simulink model "GlowPlug_harness"  (Simulink 7.7)
settings: Solver=FixedStepDiscrete  SolverMode=SingleTasking  StartTime=0.0  StopTime=100  FixedStep=0.1  RelTol=1e-3
InitFcn:
  | if signalbuilder('GlowPlug_harness/Signal_Builder','activegroup') == 1
  |   CD_GLOW_PLUG_PREHEAT_FUNCTION.DataType = 'uint8';
  |   CD_GLOW_PLUG_PREHEAT_FUNCTION.Value = 255;
  | else
  |   CD_GLOW_PLUG_PREHEAT_FUNCTION.DataType = 'uint8';
  |   CD_GLOW_PLUG_PREHEAT_FUNCTION.Value = 0;
  | end
  | 
  | if signalbuilder('GlowPlug_harness/Signal_Builder','activegroup') == 2
  |   CD_GLOW_PLUG_PREHEAT_FEEDBACK_FUNCTION.DataType = 'uint8';
  |   CD_GLOW_PLUG_PREHEAT_FEEDBACK_FUNCTION.Value = 255;
  | else
  |   CD_GLOW_PLUG_PREHEAT_FEEDBACK_FUNCTION.DataType = 'uint8';
  |   CD_GLOW_PLUG_PREHEAT_FEEDBACK_FUNCTION.Value = 0;
  | end
  | 
  | if signalbuilder('GlowPlug_harness/Signal_Builder','activegroup') == 13
  |   CD_GLOW_PLUG_OFF_WITH_LOW_BATTERY.DataType = 'uint8';
  |   CD_GLOW_PLUG_OFF_WITH_LOW_BATTERY.Value = 0;
  | elseif signalbuilder('GlowPlug_harness/Signal_Builder','activegroup') == 14
  |   CD_GLOW_PLUG_OFF_WITH_LOW_BATTERY.DataType = 'uint8';
  |   CD_GLOW_PLUG_OFF_WITH_LOW_BATTERY.Value = 0;
  | else
  |   CD_GLOW_PLUG_OFF_WITH_LOW_BATTERY.DataType = 'uint8';
  |   CD_GLOW_PLUG_OFF_WITH_LOW_BATTERY.Value = 255;
  | end
  | 
  | 
  | if signalbuilder('GlowPlug_harness/Signal_Builder','activegroup') == 1
  |   CD_GLOW_PLUG_CRANKING_FUNCTION.DataType = 'uint8';
  |   CD_GLOW_PLUG_CRANKING_FUNCTION.Value = 255;
  | else
  |   CD_GLOW_PLUG_CRANKING_FUNCTION.DataType = 'uint8';
  |   CD_GLOW_PLUG_CRANKING_FUNCTION.Value = 0;
  | end
  | 
  | if signalbuilder('GlowPlug_harness/Signal_Builder','activegroup') == 9
  |   CD_GLOW_PLUG_DEBOUNCE_CRANK.DataType = 'uint16';
  |   CD_GLOW_PLUG_DEBOUNCE_CRANK.Value = 255;
  | 
  |   UNLIMITED.DataType = 'uint16';
  |   UNLIMITED.Value = 255;
  | else
  |   CD_GLOW_PLUG_DEBOUNCE_CRANK.DataType = 'uint16';
  |   CD_GLOW_PLUG_DEBOUNCE_CRANK.Value = 300;
  | 
  |   UNLIMITED.DataType = 'uint16';
  |   UNLIMITED.Value = 65535;
  | end
  | 
  | if signalbuilder('GlowPlug_harness/Signal_Builder','activegroup') == 1
  |   CD_GLOW_PLUG_AFTERGLOW_FUNCTION.DataType = 'uint8';
  |   CD_GLOW_PLUG_AFTERGLOW_FUNCTION.Value = 255;
  | else
  |   CD_GLOW_PLUG_AFTERGLOW_FUNCTION.DataType = 'uint8';
  |   CD_GLOW_PLUG_AFTERGLOW_FUNCTION.Value = 0;
  | end
undefined symbols (not defined in the file): NON_FUNCTIONAL, OORL, sigbuilder_block, srate100
libraries: simulink x2, MX_Library x1
CloseFcn:
  | rtwprivate ssgencode ModelCloseRequest sle_main_controller
settings Model: Creator=smindema  LastModifiedBy=aliebel  CovMetricSettings=dcmtw  CovForceBlockReductionOff=off  CovCumulativeReport=on  CovModelRefEnable=off
settings MATStruct: SampleTime=0.01  Offset=0  Priority=[1.0]
settings DataIOCC: LimitDataPoints=off  SaveOutput=off  SaveTime=off
settings OptimizationCC: BlockReduction=off  InlineParams=on  ExpressionFolding=off  StateBitsets=on  DataBitsets=on  UseTempVars=on  InitFltsAndDblsToZero=on  NoFixptDivByZeroProtection=on  EfficientFloat2IntCast=on  OptimizeModelRefInitCode=on
settings DebuggingCC: SaveWithParameterizedLinksMsg=none  MultiTaskDSMMsg=warning  MultiTaskCondExecSysMsg=none  IntegerOverflowMsg=none  ModelReferenceCSMismatchMessage=warning
settings HardwareCC: ProdBitPerInt=16  ProdBitPerPointer=16  ProdIntDivRoundTo=Zero  ProdEndianess=BigEndian  ProdWordSize=16  ProdHWDeviceType=Motorola HC12
settings ModelReferenceCC: ModelReferenceNumInstancesAllowed=Single
settings RTWCC: SystemTargetFile=ert.tlc  GenCodeOnly=on  TemplateMakefile=ert_default_tmf  Description=Real-Time Workshop Embedded Coder (no auto configuration)  GenerateReport=on  RetainRTWFile=on  ProcessScript=ert_make_rtw_hook  IncludeHyperlinkInReport=on  LaunchReport=on  IncludeERTFirstTime=on
settings RTWCC: CustomHeaderCode=|
  | #include "cpp_req_defines.h"
  | #include "hw_fin.h"
  | #include "cdata.h"
settings CodeAppCC: IgnoreCustomStorageClasses=off  DefineNamingRule=UpperCase
settings ERTTargetCC: TargetFcnLib=ansi_tfl_tmw.mat  FunctionExecutionProfile=off  MultiwordLength=2048  GenerateSampleERTMain=on  IncludeMdlTerminateFcn=off  SuppressErrorStatus=on  SupportAbsoluteTime=off  SupportNonFinite=off  SupportComplex=off  PurelyIntegerCode=on  ERTCustomFileTemplate=gen_rtw_req_defines_h.tlc  GlobalDataDefinition=InSeparateSourceFile  GlobalDataReference=InSeparateHeaderFile  ConvertIfToSwitch=off

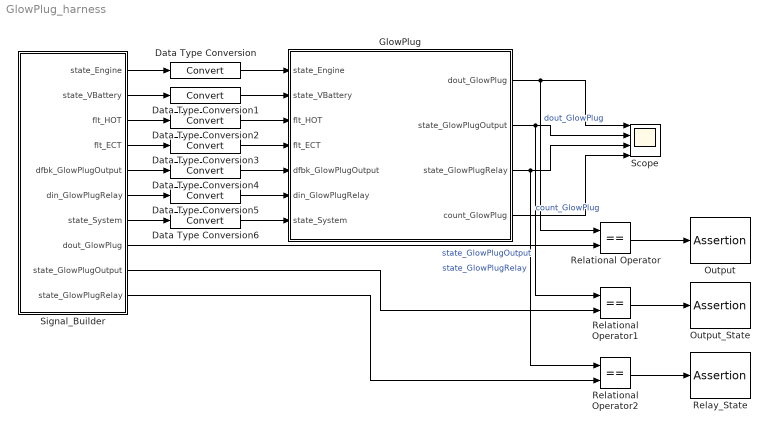
== system GlowPlug_harness ==
  Data Type Conversion{,1..6} (7 alike) : DataTypeConversion
  GlowPlug : Subsystem  TreatAsAtomicUnit=on  SystemSampleTime=srate100  RTWFileName=mod_Outputs
      settings: RTWSystemCode=Function  RTWFileNameOpts=User specified
  Output : Assertion  Enabled=off
  Output_State : Assertion  Enabled=off
  Relational Operator : RelationalOperator  Operator===  OutDataTypeStr=boolean
  Relational Operator1 : RelationalOperator  Operator===  OutDataTypeStr=boolean
  Relational Operator2 : RelationalOperator  Operator===  OutDataTypeStr=boolean
  Relay_State : Assertion  Enabled=off
  Scope : Scope  NumInputPorts=4
      settings: TimeRange=100  YMin=0~5~7~0  YMax=1~30~9~200  MaxDataPoints=50000
  Signal_Builder : Subsystem  Tag=STV Subsys  LoadFcn=sigbuilder_block('load',[166.5 143.25 1074 597.75 ]);  StartFcn=sigbuilder_block('start');  StopFcn=sigbuilder_block('stop');  ClipboardFcn=sigbuilder_block('clipboard');  mask(Sigbuilder block){}
      mask help: Create and generate interchangeable groups of signals whose waveforms are piecewise linear.
      mask init:
      | if ~strcmp(get_param(bdroot(gcbh),'SimulationStatus'),'stopped') tuvar = sigbuilder_block('maskInit'); end
      settings: CopyFcn=sigbuilder_block('copy');  DeleteFcn=sigbuilder_block('delete');  ModelCloseFcn=sigbuilder_block('modelClose');  PreSaveFcn=sigbuilder_block('preSave');  NameChangeFcn=sigbuilder_block('namechange');  OpenFcn=sigbuilder_block('open',[1274.25 150 1074 597.75 ]);  CloseFcn=sigbuilder_block('close');
      mask Display: plot(0,0,100,100,[10,10,40,40,10],[80,20,20,80,80],[40,10],[50,50], [40,27,10],[65,72,56],[40,25,25,10],[28,28,43,43]);
  wires:
  Signal_Builder/1(state_Engine) -> Data Type Conversion/1
  Data Type Conversion/1 -> GlowPlug/1(state_Engine)
  Relational Operator/1 -> Output/1
  Relational Operator1/1 -> Output_State/1
  Relational Operator2/1 -> Relay_State/1
  Signal_Builder/2(state_VBattery) -> Data Type Conversion1/1
  Signal_Builder/3(flt_HOT) -> Data Type Conversion2/1
  Signal_Builder/4(flt_ECT) -> Data Type Conversion3/1
  Signal_Builder/5(dfbk_GlowPlugOutput) -> Data Type Conversion4/1
  Signal_Builder/6(din_GlowPlugRelay) -> Data Type Conversion5/1
  Signal_Builder/7(state_System) -> Data Type Conversion6/1
  Data Type Conversion1/1 -> GlowPlug/2(state_VBattery)
  Data Type Conversion2/1 -> GlowPlug/3(flt_HOT)
  Data Type Conversion3/1 -> GlowPlug/4(flt_ECT)
  Data Type Conversion4/1 -> GlowPlug/5(dfbk_GlowPlugOutput)
  Data Type Conversion5/1 -> GlowPlug/6(din_GlowPlugRelay)
  Data Type Conversion6/1 -> GlowPlug/7(state_System)
  GlowPlug/1(dout_GlowPlug) -> Scope/1, Relational Operator/1  "dout_GlowPlug"
  GlowPlug/2(state_GlowPlugOutput) -> Scope/2, Relational Operator1/1  "state_GlowPlugOutput"
  GlowPlug/3(state_GlowPlugRelay) -> Scope/3, Relational Operator2/1  "state_GlowPlugRelay"
  GlowPlug/4(count_GlowPlug) -> Scope/4  "count_GlowPlug"
  Signal_Builder/8(dout_GlowPlug) -> Relational Operator/2
  Signal_Builder/9(state_GlowPlugOutput) -> Relational Operator1/2
  Signal_Builder/10(state_GlowPlugRelay) -> Relational Operator2/2

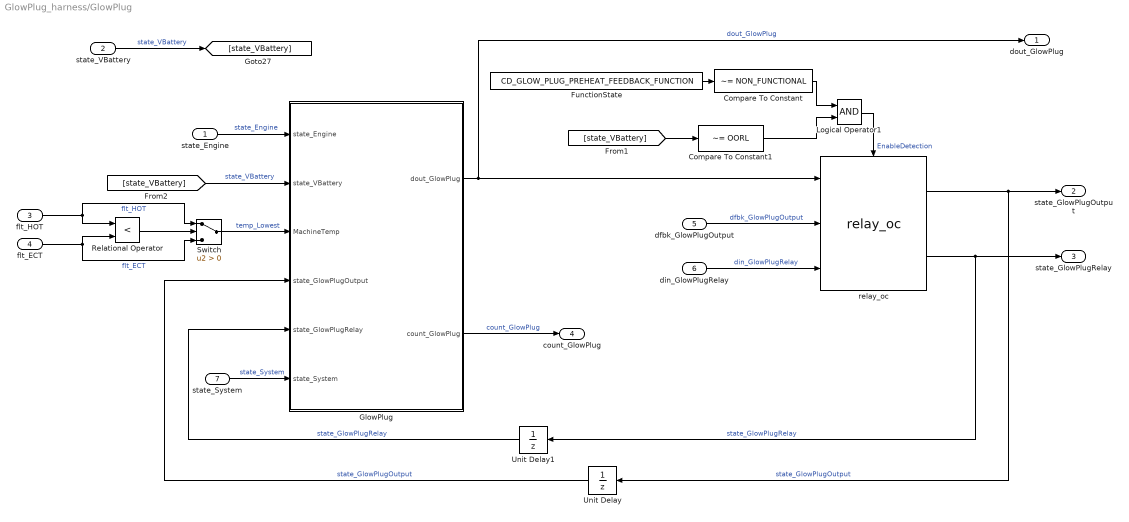
== system GlowPlug_harness/GlowPlug ==
  state_Engine : Inport
  state_VBattery : Inport  Port=2
  flt_HOT : Inport  Port=3
  flt_ECT : Inport  Port=4
  dfbk_GlowPlugOutput : Inport  Port=5
  din_GlowPlugRelay : Inport  Port=6
  state_System : Inport  Port=7
  Compare To Constant : simulink/Logic and Bit Operations/Compare To Constant  SystemSampleTime=-1  relop=~=  const=NON_FUNCTIONAL  LogicOutDataTypeMode=boolean  ZeroCross=off
  Compare To Constant1 : simulink/Logic and Bit Operations/Compare To Constant  SystemSampleTime=-1  relop=~=  const=OORL  LogicOutDataTypeMode=boolean  ZeroCross=off
  FunctionState : Constant  Value=CD_GLOW_PLUG_PREHEAT_FEEDBACK_FUNCTION  OutDataTypeStr=uint8
  GlowPlug : Stateflow chart  TreatAsAtomicUnit=on
  Logical Operator1 : Logic  AllPortsSameDT=off  OutDataTypeStr=boolean
  Relational Operator : RelationalOperator  Operator=<  OutDataTypeStr=boolean  ZeroCross=off
  Switch : Switch  Criteria=u2 > Threshold  ZeroCross=off
  Unit Delay : UnitDelay  X0=8  SampleTime=-1
      settings: AttributesFormatString=<initial=%<X0>>\n<tsample=%<SampleTime>>
  Unit Delay1 : UnitDelay  X0=8  SampleTime=-1
      settings: AttributesFormatString=<initial=%<X0>>\n<tsample=%<SampleTime>>
  relay_oc : MX_Library/relay_oc  SystemSampleTime=-1  ERROR_ON_DB_CNT=CD_GLOW_PLUG_DEBOUNCE_ERROR_ON  ERROR_OFF_DB_CNT=CD_GLOW_PLUG_DEBOUNCE_ERROR_OFF  NORMAL_DB_CNT=CD_GLOW_PLUG_DEBOUNCE_NORMAL
  dout_GlowPlug : Outport
  state_GlowPlugOutput : Outport  Port=2
  state_GlowPlugRelay : Outport  Port=3
  count_GlowPlug : Outport  Port=4
  wires:
  [state_VBattery] -> GlowPlug/2(state_VBattery)  "state_VBattery"
  Switch/1 -> GlowPlug/3(MachineTemp)  "temp_Lowest"
  flt_HOT/1 -> Switch/1, Relational Operator/1  "flt_HOT"
  flt_ECT/1 -> Switch/3, Relational Operator/2  "flt_ECT"
  Relational Operator/1 -> Switch/2
  state_System/1 -> GlowPlug/6(state_System)  "state_System"
  GlowPlug/2(count_GlowPlug) -> count_GlowPlug/1  "count_GlowPlug"
  state_VBattery/1 -> [state_VBattery]  "state_VBattery"
  Logical Operator1/1 -> relay_oc/Enable  "EnableDetection"
  Compare To Constant1/1 -> Logical Operator1/2
  Compare To Constant/1 -> Logical Operator1/1
  [state_VBattery] -> Compare To Constant1/1
  FunctionState/1 -> Compare To Constant/1
  Unit Delay1/1 -> GlowPlug/5(state_GlowPlugRelay)  "state_GlowPlugRelay"
  Unit Delay/1 -> GlowPlug/4(state_GlowPlugOutput)  "state_GlowPlugOutput"
  GlowPlug/1(dout_GlowPlug) -> dout_GlowPlug/1, relay_oc/1  "dout_GlowPlug"
  state_Engine/1 -> GlowPlug/1(state_Engine)  "state_Engine"
  din_GlowPlugRelay/1 -> relay_oc/3  "din_GlowPlugRelay"
  dfbk_GlowPlugOutput/1 -> relay_oc/2  "dfbk_GlowPlugOutput"
  relay_oc/2 -> Unit Delay1/1, state_GlowPlugRelay/1  "state_GlowPlugRelay"
  relay_oc/1 -> Unit Delay/1, state_GlowPlugOutput/1  "state_GlowPlugOutput"

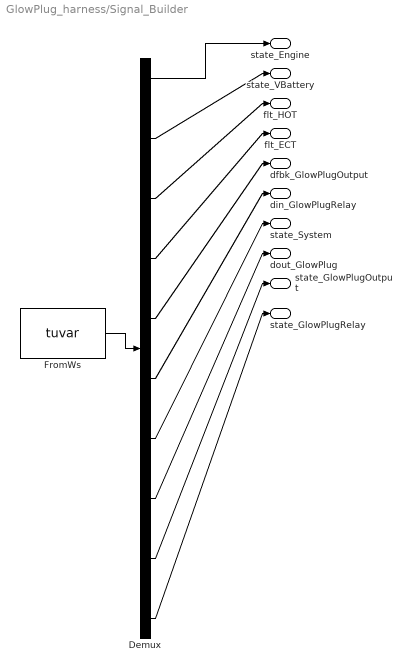
== system GlowPlug_harness/Signal_Builder ==
  Demux : Demux  Tag=STV Demux  Outputs=10
  FromWs : FromWorkspace  Tag=STV FromWs  VariableName=tuvar  SampleTime=0  SigBuilderData=DataTag0  VnvData=DataTag1
      SigBuilderData=|
      | common.afterFinalStr = 'Extrapolate'
      | common.sampleTime = 0
      | dataSet(1).timeRange = [0 100]
      | dataSet(1).name = 'T1_Nonfunc'
      | dataSet(2).timeRange = [0 100]
      | dataSet(2).name = 'T2-No_Feedback'
      | dataSet(3).timeRange = [0 100]
      | dataSet(3).name = 'T3-Level0'
      | dataSet(4).timeRange = [0 100]
      | dataSet(4).name = 'T4-Level1'
      | dataSet(5).timeRange = [0 100]
      | dataSet(5).name = 'T5-Level2'
      | dataSet(6).timeRange = [0 100]
      | dataSet(6).name = 'T6-Level3'
      | dataSet(7).timeRange = [0 100]
      | dataSet(7).name = 'T7-Out_ErrOnOff'
      | dataSet(8).timeRange = [0 100]
      | dataSet(8).name = 'T8-Relay_ErrOnOff'
      | dataSet(9).timeRange = [0 100]
      | dataSet(9).name = 'T9-Out_OC_Failure'
      | dataSet(10).timeRange = [0 100]
      | dataSet(10).name = 'T10-Afterglow_Failure'
      | dataSet(11).timeRange = [0 100]
      | dataSet(11).name = 'T11-Failure2'
      | dataSet(12).timeRange = [0 100]
      | dataSet(12).name = 'T12-System'
      | dataSet(13).timeRange = [0 100]
      | dataSet(13).name = 'T13-Voltage'
      | dataSet(14).timeRange = [0 100]
      | dataSet(14).name = 'T14-Voltage2'
      | dataSet(15).timeRange = [0 100]
      | dataSet(15).name = 'T15-ErrorOn'
      | sbobj.Groups(1).Name = 'T1_Nonfunc'
      | sbobj.Groups(1).Signals(1).Name = 'state_Engine'
      | sbobj.Groups(1).Signals(1).XData = [0 39.9 39.9 50.1 50.1 59.9 59.9 100]
      | sbobj.Groups(1).Signals(1).YData = [1 1 2 2 3 3 1 1]
      | sbobj.Groups(1).Signals(2).Name = 'state_VBattery'
      | sbobj.Groups(1).Signals(2).XData = [0 100]
      | sbobj.Groups(1).Signals(2).YData = [8 8]
      | sbobj.Groups(1).Signals(3).Name = 'flt_HOT'
      | sbobj.Groups(1).Signals(3).XData = [0 100]
      | sbobj.Groups(1).Signals(3).YData = [50 50]
      | sbobj.Groups(1).Signals(4).Name = 'flt_ECT'
      | sbobj.Groups(1).Signals(4).XData = [0 100]
      | sbobj.Groups(1).Signals(4).YData = [40 40]
      | sbobj.Groups(1).Signals(5).Name = 'dfbk_GlowPlugOutput'
      | sbobj.Groups(1).Signals(5).XData = [0 100]
      | sbobj.Groups(1).Signals(5).YData = [0 0]
      | sbobj.Groups(1).Signals(6).Name = 'din_GlowPlugRelay'
      | sbobj.Groups(1).Signals(6).XData = [0 100]
      | sbobj.Groups(1).Signals(6).YData = [0 0]
      | sbobj.Groups(1).Signals(7).Name = 'state_System'
      | sbobj.Groups(1).Signals(7).XData = [0 20 20 100]
      | sbobj.Groups(1).Signals(7).YData = [1 1 0 0]
      | sbobj.Groups(1).Signals(8).Name = 'dout_GlowPlug'
      | sbobj.Groups(1).Signals(8).XData = [0 100]
      | sbobj.Groups(1).Signals(8).YData = [0 0]
      | sbobj.Groups(1).Signals(9).Name = 'state_GlowPlugOutput'
      | sbobj.Groups(1).Signals(9).XData = [0 100]
      | sbobj.Groups(1).Signals(9).YData = [8 8]
      | sbobj.Groups(1).Signals(10).Name = 'state_GlowPlugRelay'
      | sbobj.Groups(1).Signals(10).XData = [0 100]
      | sbobj.Groups(1).Signals(10).YData = [8 8]
      | sbobj.Groups(2).Name = 'T2-No_Feedback'
      | sbobj.Groups(2).Signals(1).Name = 'state_Engine'
      | sbobj.Groups(2).Signals(1).XData = [0 10 10 50.2 50.2 100]
      | sbobj.Groups(2).Signals(1).YData = [1 1 2 2 1 1]
      | sbobj.Groups(2).Signals(2).Name = 'state_VBattery'
      | sbobj.Groups(2).Signals(2).XData = [0 100]
      | sbobj.Groups(2).Signals(2).YData = [8 8]
      | sbobj.Groups(2).Signals(3).Name = 'flt_HOT'
      | sbobj.Groups(2).Signals(3).XData = [0 100]
      | sbobj.Groups(2).Signals(3).YData = [50 50]
      | sbobj.Groups(2).Signals(4).Name = 'flt_ECT'
      | sbobj.Groups(2).Signals(4).XData = [0 100]
      | sbobj.Groups(2).Signals(4).YData = [40 40]
      | sbobj.Groups(2).Signals(5).Name = 'dfbk_GlowPlugOutput'
      | sbobj.Groups(2).Signals(5).XData = [0 100]
      | sbobj.Groups(2).Signals(5).YData = [0 0]
      | sbobj.Groups(2).Signals(6).Name = 'din_GlowPlugRelay'
      | sbobj.Groups(2).Signals(6).XData = [0 5.4 5.4 100]
      | sbobj.Groups(2).Signals(6).YData = [1 1 0 0]
      | sbobj.Groups(2).Signals(7).Name = 'state_System'
      | sbobj.Groups(2).Signals(7).XData = [0 100]
      | sbobj.Groups(2).Signals(7).YData = [1 1]
      | sbobj.Groups(2).Signals(8).Name = 'dout_GlowPlug'
      | sbobj.Groups(2).Signals(8).XData = [0 0.6 0.6 10 10 10.1 10.1 40.2 40.2 100]
      | sbobj.Groups(2).Signals(8).YData = [0 0 1 1 0 0 1 1 0 0]
      | sbobj.Groups(2).Signals(9).Name = 'state_GlowPlugOutput'
      | sbobj.Groups(2).Signals(9).XData = [0 100]
      | sbobj.Groups(2).Signals(9).YData = [8 8]
      | sbobj.Groups(2).Signals(10).Name = 'state_GlowPlugRelay'
      | sbobj.Groups(2).Signals(10).XData = [0 100]
      | sbobj.Groups(2).Signals(10).YData = [8 8]
      | sbobj.Groups(3).Name = 'T3-Level0'
      | sbobj.Groups(3).Signals(1).Name = 'state_Engine'
      | sbobj.Groups(3).Signals(1).XData = [0 67 67 71.1 71.1 100]
      | sbobj.Groups(3).Signals(1).YData = [1 1 2 2 3 3]
      | sbobj.Groups(3).Signals(2).Name = 'state_VBattery'
      | sbobj.Groups(3).Signals(2).XData = [0 100]
      | sbobj.Groups(3).Signals(2).YData = [8 8]
      | sbobj.Groups(3).Signals(3).Name = 'flt_HOT'
      | sbobj.Groups(3).Signals(3).XData = [0 100]
      | sbobj.Groups(3).Signals(3).YData = [50 50]
      | sbobj.Groups(3).Signals(4).Name = 'flt_ECT'
      | sbobj.Groups(3).Signals(4).XData = [0 100]
      | sbobj.Groups(3).Signals(4).YData = [40 40]
      | sbobj.Groups(3).Signals(5).Name = 'dfbk_GlowPlugOutput'
      | sbobj.Groups(3).Signals(5).XData = [0 0.8 0.8 30.7 30.7 35.9 35.9 66 66 67 67 80.9 80.9 100]
      | sbobj.Groups(3).Signals(5).YData = [0 0 1 1 0 0 1 1 0 0 1 1 0 0]
      | sbobj.Groups(3).Signals(6).Name = 'din_GlowPlugRelay'
      | sbobj.Groups(3).Signals(6).XData = [0 0.8 0.8 30.5 30.5 35.7 35.7 66 66 67 67 81 81 100]
      | sbobj.Groups(3).Signals(6).YData = [0 0 1 1 0 0 1 1 0 0 1 1 0 0]
      | sbobj.Groups(3).Signals(7).Name = 'state_System'
      | sbobj.Groups(3).Signals(7).XData = [0 100]
      | sbobj.Groups(3).Signals(7).YData = [1 1]
      | sbobj.Groups(3).Signals(8).Name = 'dout_GlowPlug'
      | sbobj.Groups(3).Signals(8).XData = [0 0.6 0.6 30.7 30.7 35.8 35.8 65.9 65.9 67 67 71.1 71.1 71.2 71.2 81.3 81.3 100]
      | sbobj.Groups(3).Signals(8).YData = [0 0 1 1 0 0 1 1 0 0 1 1 0 0 1 1 0 0]
      | sbobj.Groups(3).Signals(9).Name = 'state_GlowPlugOutput'
      | sbobj.Groups(3).Signals(9).XData = [0 100]
      | sbobj.Groups(3).Signals(9).YData = [8 8]
      | sbobj.Groups(3).Signals(10).Name = 'state_GlowPlugRelay'
      | sbobj.Groups(3).Signals(10).XData = [0 100]
      | sbobj.Groups(3).Signals(10).YData = [8 8]
      | sbobj.Groups(4).Name = 'T4-Level1'
      | sbobj.Groups(4).Signals(1).Name = 'state_Engine'
      | sbobj.Groups(4).Signals(1).XData = [0 60 60 65 65 100]
      | sbobj.Groups(4).Signals(1).YData = [1 1 2 2 3 3]
      | sbobj.Groups(4).Signals(2).Name = 'state_VBattery'
      | sbobj.Groups(4).Signals(2).XData = [0 100]
      | sbobj.Groups(4).Signals(2).YData = [8 8]
      | sbobj.Groups(4).Signals(3).Name = 'flt_HOT'
      | sbobj.Groups(4).Signals(3).XData = [0 100]
      | sbobj.Groups(4).Signals(3).YData = [70 70]
      | sbobj.Groups(4).Signals(4).Name = 'flt_ECT'
      | sbobj.Groups(4).Signals(4).XData = [0 100]
      | sbobj.Groups(4).Signals(4).YData = [90 90]
      | sbobj.Groups(4).Signals(5).Name = 'dfbk_GlowPlugOutput'
      | sbobj.Groups(4).Signals(5).XData = [0 1.4 1.4 21.5 21.5 26.6 26.6 46.6 46.6 60 60 65 65 65.1 65.1 70.7 70.7 100]
      | sbobj.Groups(4).Signals(5).YData = [0 0 1 1 0 0 1 1 0 0 1 1 0 0 1 1 0 0]
      | sbobj.Groups(4).Signals(6).Name = 'din_GlowPlugRelay'
      | sbobj.Groups(4).Signals(6).XData = [0 1.4 1.4 21.5 21.5 26.6 26.6 46.7 46.7 60 60 71 71 100]
      | sbobj.Groups(4).Signals(6).YData = [0 0 1 1 0 0 1 1 0 0 1 1 0 0]
      | sbobj.Groups(4).Signals(7).Name = 'state_System'
      | sbobj.Groups(4).Signals(7).XData = [0 100]
      | sbobj.Groups(4).Signals(7).YData = [1 1]
      | sbobj.Groups(4).Signals(8).Name = 'dout_GlowPlug'
      | sbobj.Groups(4).Signals(8).XData = [0 0.6 0.6 20.7 20.7 25.8 25.8 45.9 45.9 60 60 65 65 65.1 65.1 71.2 71.2 100]
      | sbobj.Groups(4).Signals(8).YData = [0 0 1 1 0 0 1 1 0 0 1 1 0 0 1 1 0 0]
      | sbobj.Groups(4).Signals(9).Name = 'state_GlowPlugOutput'
      | sbobj.Groups(4).Signals(9).XData = [0 100]
      | sbobj.Groups(4).Signals(9).YData = [8 8]
      | sbobj.Groups(4).Signals(10).Name = 'state_GlowPlugRelay'
      | sbobj.Groups(4).Signals(10).XData = [0 100]
      | sbobj.Groups(4).Signals(10).YData = [8 8]
      | sbobj.Groups(5).Name = 'T5-Level2'
      | sbobj.Groups(5).Signals(1).Name = 'state_Engine'
      | sbobj.Groups(5).Signals(1).XData = [0 50 50 52.4 52.4 100]
      | sbobj.Groups(5).Signals(1).YData = [1 1 2 2 3 3]
      | sbobj.Groups(5).Signals(2).Name = 'state_VBattery'
      | sbobj.Groups(5).Signals(2).XData = [0 100]
      | sbobj.Groups(5).Signals(2).YData = [8 8]
      | sbobj.Groups(5).Signals(3).Name = 'flt_HOT'
      | sbobj.Groups(5).Signals(3).XData = [0 100]
      | sbobj.Groups(5).Signals(3).YData = [80 80]
      | sbobj.Groups(5).Signals(4).Name = 'flt_ECT'
      | sbobj.Groups(5).Signals(4).XData = [0 100]
      | sbobj.Groups(5).Signals(4).YData = [120 120]
      | sbobj.Groups(5).Signals(5).Name = 'dfbk_GlowPlugOutput'
      | sbobj.Groups(5).Signals(5).XData = [0 0.8 0.8 10.5 10.5 15.5 15.5 26.1 26.1 50 50 54.9 54.9 100]
      | sbobj.Groups(5).Signals(5).YData = [0 0 1 1 0 0 1 1 0 0 1 1 0 0]
      | sbobj.Groups(5).Signals(6).Name = 'din_GlowPlugRelay'
      | sbobj.Groups(5).Signals(6).XData = [0 0.8 0.8 10.5 10.5 15.4 15.4 25.8 25.8 50 50 54.7 54.7 100]
      | sbobj.Groups(5).Signals(6).YData = [0 0 1 1 0 0 1 1 0 0 1 1 0 0]
      | sbobj.Groups(5).Signals(7).Name = 'state_System'
      | sbobj.Groups(5).Signals(7).XData = [0 100]
      | sbobj.Groups(5).Signals(7).YData = [1 1]
      | sbobj.Groups(5).Signals(8).Name = 'dout_GlowPlug'
      | sbobj.Groups(5).Signals(8).XData = [0 0.6 0.6 10.7 10.7 15.8 15.8 25.9 25.9 50 50 52.4 52.4 52.5 52.5 54.6 54.6 100]
      | sbobj.Groups(5).Signals(8).YData = [0 0 1 1 0 0 1 1 0 0 1 1 0 0 1 1 0 0]
      | sbobj.Groups(5).Signals(9).Name = 'state_GlowPlugOutput'
      | sbobj.Groups(5).Signals(9).XData = [0 100]
      | sbobj.Groups(5).Signals(9).YData = [8 8]
      | sbobj.Groups(5).Signals(10).Name = 'state_GlowPlugRelay'
      | sbobj.Groups(5).Signals(10).XData = [0 100]
      | sbobj.Groups(5).Signals(10).YData = [8 8]
      | sbobj.Groups(6).Name = 'T6-Level3'
      | sbobj.Groups(6).Signals(1).Name = 'state_Engine'
      | sbobj.Groups(6).Signals(1).XData = [0 40 40 74.6 74.6 100]
      | sbobj.Groups(6).Signals(1).YData = [1 1 2 2 3 3]
      | sbobj.Groups(6).Signals(2).Name = 'state_VBattery'
      | sbobj.Groups(6).Signals(2).XData = [0 100]
      | sbobj.Groups(6).Signals(2).YData = [8 8]
      | sbobj.Groups(6).Signals(3).Name = 'flt_HOT'
      | sbobj.Groups(6).Signals(3).XData = [0 100]
      | sbobj.Groups(6).Signals(3).YData = [140 140]
      | sbobj.Groups(6).Signals(4).Name = 'flt_ECT'
      | sbobj.Groups(6).Signals(4).XData = [0 100]
      | sbobj.Groups(6).Signals(4).YData = [110 110]
      | sbobj.Groups(6).Signals(5).Name = 'dfbk_GlowPlugOutput'
      | sbobj.Groups(6).Signals(5).XData = [0 40 40 70.1 70.1 74.6 74.6 74.8 74.8 100]
      | sbobj.Groups(6).Signals(5).YData = [0 0 1 1 0 0 1 1 0 0]
      | sbobj.Groups(6).Signals(6).Name = 'din_GlowPlugRelay'
      | sbobj.Groups(6).Signals(6).XData = [0 39.9 39.9 70.1 70.1 74.7 74.7 74.8 74.8 100]
      | sbobj.Groups(6).Signals(6).YData = [0 0 1 1 0 0 1 1 0 0]
      | sbobj.Groups(6).Signals(7).Name = 'state_System'
      | sbobj.Groups(6).Signals(7).XData = [0 100]
      | sbobj.Groups(6).Signals(7).YData = [1 1]
      | sbobj.Groups(6).Signals(8).Name = 'dout_GlowPlug'
      | sbobj.Groups(6).Signals(8).XData = [0 40 40 70.1 70.1 74.6 74.6 74.7 74.7 100]
      | sbobj.Groups(6).Signals(8).YData = [0 0 1 1 0 0 1 1 0 0]
      | sbobj.Groups(6).Signals(9).Name = 'state_GlowPlugOutput'
      | sbobj.Groups(6).Signals(9).XData = [0 100]
      | sbobj.Groups(6).Signals(9).YData = [8 8]
      | sbobj.Groups(6).Signals(10).Name = 'state_GlowPlugRelay'
      | sbobj.Groups(6).Signals(10).XData = [0 100]
      | sbobj.Groups(6).Signals(10).YData = [8 8]
      | sbobj.Groups(7).Name = 'T7-Out_ErrOnOff'
      | sbobj.Groups(7).Signals(1).Name = 'state_Engine'
      | sbobj.Groups(7).Signals(1).XData = [0 0.1 0.1 9.2 9.2 13.9 13.9 100]
      | sbobj.Groups(7).Signals(1).YData = [1 1 2 2 3 3 1 1]
      | sbobj.Groups(7).Signals(2).Name = 'state_VBattery'
      | sbobj.Groups(7).Signals(2).XData = [0 100]
      | sbobj.Groups(7).Signals(2).YData = [8 8]
      | sbobj.Groups(7).Signals(3).Name = 'flt_HOT'
      | sbobj.Groups(7).Signals(3).XData = [0 100]
      | sbobj.Groups(7).Signals(3).YData = [140 140]
      | sbobj.Groups(7).Signals(4).Name = 'flt_ECT'
      | sbobj.Groups(7).Signals(4).XData = [0 100]
      | sbobj.Groups(7).Signals(4).YData = [120 120]
      | sbobj.Groups(7).Signals(5).Name = 'dfbk_GlowPlugOutput'
      | sbobj.Groups(7).Signals(5).XData = [0 36.5 36.5 69.2 69.2 100]
      | sbobj.Groups(7).Signals(5).YData = [0 0 1 1 0 0]
      | sbobj.Groups(7).Signals(6).Name = 'din_GlowPlugRelay'
      | sbobj.Groups(7).Signals(6).XData = [0 36.4 36.4 69.2 69.2 100]
      | sbobj.Groups(7).Signals(6).YData = [0 0 1 1 0 0]
      | sbobj.Groups(7).Signals(7).Name = 'state_System'
      | sbobj.Groups(7).Signals(7).XData = [0 100]
      | sbobj.Groups(7).Signals(7).YData = [1 1]
      | sbobj.Groups(7).Signals(8).Name = 'dout_GlowPlug'
      | sbobj.Groups(7).Signals(8).XData = [0 0.6 0.6 0.7 5.8 5.8 100]
      | sbobj.Groups(7).Signals(8).YData = [0 0 1 1 1 0 0]
      | sbobj.Groups(7).Signals(9).Name = 'state_GlowPlugOutput'
      | sbobj.Groups(7).Signals(9).XData = [0 5.7 5.7 20.9 20.9 66.6 66.6 84.3 84.3 100]
      | sbobj.Groups(7).Signals(9).YData = [8 8 3 3 8 8 2 2 8 8]
      | sbobj.Groups(7).Signals(10).Name = 'state_GlowPlugRelay'
      | sbobj.Groups(7).Signals(10).XData = [0 100]
      | sbobj.Groups(7).Signals(10).YData = [8 8]
      | sbobj.Groups(8).Name = 'T8-Relay_ErrOnOff'
      | sbobj.Groups(8).Signals(1).Name = 'state_Engine'
      | sbobj.Groups(8).Signals(1).XData = [0 35 35 37.6 37.6 41.1 41.1 70.2 70.2 89.8 89.8 94.4 94.4 96.9 96.9 100]
      | sbobj.Groups(8).Signals(1).YData = [1 1 2 2 3 3 1 1 2 2 1 1 2 2 1 1]
      | sbobj.Groups(8).Signals(2).Name = 'state_VBattery'
      | sbobj.Groups(8).Signals(2).XData = [0 92.9 92.9 100]
      | sbobj.Groups(8).Signals(2).YData = [8 8 22 22]
      | sbobj.Groups(8).Signals(3).Name = 'flt_HOT'
      | sbobj.Groups(8).Signals(3).XData = [0 100]
      | sbobj.Groups(8).Signals(3).YData = [140 140]
      | sbobj.Groups(8).Signals(4).Name = 'flt_ECT'
      | sbobj.Groups(8).Signals(4).XData = [0 100]
      | sbobj.Groups(8).Signals(4).YData = [110 110]
      | sbobj.Groups(8).Signals(5).Name = 'dfbk_GlowPlugOutput'
      | sbobj.Groups(8).Signals(5).XData = [0 40 70.2 70.2 90 90 100]
      | sbobj.Groups(8).Signals(5).YData = [0 0 0 1 1 0 0]
      | sbobj.Groups(8).Signals(6).Name = 'din_GlowPlugRelay'
      | sbobj.Groups(8).Signals(6).XData = [0 40 40 100]
      | sbobj.Groups(8).Signals(6).YData = [1 1 0 0]
      | sbobj.Groups(8).Signals(7).Name = 'state_System'
      | sbobj.Groups(8).Signals(7).XData = [0 100]
      | sbobj.Groups(8).Signals(7).YData = [1 1]
      | sbobj.Groups(8).Signals(8).Name = 'dout_GlowPlug'
      | sbobj.Groups(8).Signals(8).XData = [0 70.2 70.2 75.4 75.4 100]
      | sbobj.Groups(8).Signals(8).YData = [0 0 1 1 0 0]
      | sbobj.Groups(8).Signals(9).Name = 'state_GlowPlugOutput'
      | sbobj.Groups(8).Signals(9).XData = [0 30.2 55.1 75.2 90.4 100]
      | sbobj.Groups(8).Signals(9).YData = [8 8 8 8 8 8]
      | sbobj.Groups(8).Signals(10).Name = 'state_GlowPlugRelay'
      | sbobj.Groups(8).Signals(10).XData = [0 30.2 30.2 55.1 55.1 75.3 75.3 90.5 90.5 100]
      | sbobj.Groups(8).Signals(10).YData = [8 8 2 2 8 8 3 3 8 8]
      | sbobj.Groups(9).Name = 'T9-Out_OC_Failure'
      | sbobj.Groups(9).Signals(1).Name = 'state_Engine'
      | sbobj.Groups(9).Signals(1).XData = [0 10 10 20 20 23.3 23.3 78.8 78.8 82.6 82.6 96 100]
      | sbobj.Groups(9).Signals(1).YData = [1 1 2 2 3 3 1 1 2 2 1 1 1]
      | sbobj.Groups(9).Signals(2).Name = 'state_VBattery'
      | sbobj.Groups(9).Signals(2).XData = [0 100]
      | sbobj.Groups(9).Signals(2).YData = [8 8]
      | sbobj.Groups(9).Signals(3).Name = 'flt_HOT'
      | sbobj.Groups(9).Signals(3).XData = [0 100]
      | sbobj.Groups(9).Signals(3).YData = [140 140]
      | sbobj.Groups(9).Signals(4).Name = 'flt_ECT'
      | sbobj.Groups(9).Signals(4).XData = [0 100]
      | sbobj.Groups(9).Signals(4).YData = [60 60]
      | sbobj.Groups(9).Signals(5).Name = 'dfbk_GlowPlugOutput'
      | sbobj.Groups(9).Signals(5).XData = [0 40 60 60 68.7 68.7 100]
      | sbobj.Groups(9).Signals(5).YData = [0 0 0 1 1 0 0]
      | sbobj.Groups(9).Signals(6).Name = 'din_GlowPlugRelay'
      | sbobj.Groups(9).Signals(6).XData = [0 23.2 23.2 100]
      | sbobj.Groups(9).Signals(6).YData = [1 1 0 0]
      | sbobj.Groups(9).Signals(7).Name = 'state_System'
      | sbobj.Groups(9).Signals(7).XData = [0 100]
      | sbobj.Groups(9).Signals(7).YData = [1 1]
      | sbobj.Groups(9).Signals(8).Name = 'dout_GlowPlug'
      | sbobj.Groups(9).Signals(8).XData = [0 0.6 0.6 10 10 10.1 10.1 20 20 20.1 20.1 26.2 26.2 100]
      | sbobj.Groups(9).Signals(8).YData = [0 0 1 1 0 0 1 1 0 0 1 1 0 0]
      | sbobj.Groups(9).Signals(9).Name = 'state_GlowPlugOutput'
      | sbobj.Groups(9).Signals(9).XData = [0 5.7 5.7 41.3 41.3 65.1 65.1 83.8 83.8 100]
      | sbobj.Groups(9).Signals(9).YData = [8 8 28 28 8 8 7 7 8 8]
      | sbobj.Groups(9).Signals(10).Name = 'state_GlowPlugRelay'
      | sbobj.Groups(9).Signals(10).XData = [0 100]
      | sbobj.Groups(9).Signals(10).YData = [8 8]
      | sbobj.Groups(10).Name = 'T10-Afterglow_Failure'
      | sbobj.Groups(10).Signals(1).Name = 'state_Engine'
      | sbobj.Groups(10).Signals(1).XData = [0 10 10 20.1 20.1 30 30 59.9 59.9 64.1 64.1 83.3 83.3 100]
      | sbobj.Groups(10).Signals(1).YData = [1 1 2 2 3 3 1 1 2 2 3 3 1 1]
      | sbobj.Groups(10).Signals(2).Name = 'state_VBattery'
      | sbobj.Groups(10).Signals(2).XData = [0 100]
      | sbobj.Groups(10).Signals(2).YData = [8 8]
      | sbobj.Groups(10).Signals(3).Name = 'flt_HOT'
      | sbobj.Groups(10).Signals(3).XData = [0 100]
      | sbobj.Groups(10).Signals(3).YData = [140 140]
      | sbobj.Groups(10).Signals(4).Name = 'flt_ECT'
      | sbobj.Groups(10).Signals(4).XData = [0 100]
      | sbobj.Groups(10).Signals(4).YData = [60 60]
      | sbobj.Groups(10).Signals(5).Name = 'dfbk_GlowPlugOutput'
      | sbobj.Groups(10).Signals(5).XData = [0 59.9 59.9 72.4 72.4 100]
      | sbobj.Groups(10).Signals(5).YData = [0 0 1 1 0 0]
      | sbobj.Groups(10).Signals(6).Name = 'din_GlowPlugRelay'
      | sbobj.Groups(10).Signals(6).XData = [0 30.1 30.1 100]
      | sbobj.Groups(10).Signals(6).YData = [1 1 0 0]
      | sbobj.Groups(10).Signals(7).Name = 'state_System'
      | sbobj.Groups(10).Signals(7).XData = [0 100]
      | sbobj.Groups(10).Signals(7).YData = [1 1]
      | sbobj.Groups(10).Signals(8).Name = 'dout_GlowPlug'
      | sbobj.Groups(10).Signals(8).XData = [0 0.6 0.6 10 10 10.1 10.1 20.1 20.1 20.2 20.2 26.3 26.3 59.9 59.9 64.1 64.1 64.2 64.2 69.4 69.4 100]
      | sbobj.Groups(10).Signals(8).YData = [0 0 1 1 0 0 1 1 0 0 1 1 0 0 1 1 0 0 1 1 0 0]
      | sbobj.Groups(10).Signals(9).Name = 'state_GlowPlugOutput'
      | sbobj.Groups(10).Signals(9).XData = [0 5.7 5.7 41.4 41.4 69.3 99.5 100]
      | sbobj.Groups(10).Signals(9).YData = [8 8 28 28 8 8 8 8]
      | sbobj.Groups(10).Signals(10).Name = 'state_GlowPlugRelay'
      | sbobj.Groups(10).Signals(10).XData = [0 69.3 69.3 84.5 84.5 100]
      | sbobj.Groups(10).Signals(10).YData = [8 8 3 3 8 8]
      | sbobj.Groups(11).Name = 'T11-Failure2'
      | sbobj.Groups(11).Signals(1).Name = 'state_Engine'
      | sbobj.Groups(11).Signals(1).XData = [0 10 10 25.2 25.2 51.4 51.4 60 60 73.2 73.2 78.8 78.8 82.6 82.6 100]
      | sbobj.Groups(11).Signals(1).YData = [4 4 2 2 1 1 2 2 3 3 1 1 3 3 1 1]
      | sbobj.Groups(11).Signals(2).Name = 'state_VBattery'
      | sbobj.Groups(11).Signals(2).XData = [0 100]
      | sbobj.Groups(11).Signals(2).YData = [8 8]
      | sbobj.Groups(11).Signals(3).Name = 'flt_HOT'
      | sbobj.Groups(11).Signals(3).XData = [0 100]
      | sbobj.Groups(11).Signals(3).YData = [140 140]
      | sbobj.Groups(11).Signals(4).Name = 'flt_ECT'
      | sbobj.Groups(11).Signals(4).XData = [0 100]
      | sbobj.Groups(11).Signals(4).YData = [40 40]
      | sbobj.Groups(11).Signals(5).Name = 'dfbk_GlowPlugOutput'
      | sbobj.Groups(11).Signals(5).XData = [0 24.1 24.1 44.1 44.1 49 49 51.4 51.4 60 60 70.4 70.4 100]
      | sbobj.Groups(11).Signals(5).YData = [0 0 1 1 0 0 1 1 0 0 1 1 0 0]
      | sbobj.Groups(11).Signals(6).Name = 'din_GlowPlugRelay'
      | sbobj.Groups(11).Signals(6).XData = [0 44.2 44.2 49 49 51.4 51.4 100]
      | sbobj.Groups(11).Signals(6).YData = [1 1 0 0 1 1 0 0]
      | sbobj.Groups(11).Signals(7).Name = 'state_System'
      | sbobj.Groups(11).Signals(7).XData = [0 100]
      | sbobj.Groups(11).Signals(7).YData = [1 1]
      | sbobj.Groups(11).Signals(8).Name = 'dout_GlowPlug'
      | sbobj.Groups(11).Signals(8).XData = [0 10 10 25.2 25.2 25.3 25.3 51.4 51.4 60 60 65.2 65.2 100]
      | sbobj.Groups(11).Signals(8).YData = [0 0 1 1 0 0 1 1 0 0 1 1 0 0]
      | sbobj.Groups(11).Signals(9).Name = 'state_GlowPlugOutput'
      | sbobj.Groups(11).Signals(9).XData = [0 15.1 15.1 40.4 40.4 100]
      | sbobj.Groups(11).Signals(9).YData = [8 8 28 28 8 8]
      | sbobj.Groups(11).Signals(10).Name = 'state_GlowPlugRelay'
      | sbobj.Groups(11).Signals(10).XData = [0 65.1 65.1 80.3 80.3 100]
      | sbobj.Groups(11).Signals(10).YData = [8 8 3 3 8 8]
      | sbobj.Groups(12).Name = 'T12-System'
      | sbobj.Groups(12).Signals(1).Name = 'state_Engine'
      | sbobj.Groups(12).Signals(1).XData = [0 67 67 71.1 71.1 100]
      | sbobj.Groups(12).Signals(1).YData = [1 1 2 2 3 3]
      | sbobj.Groups(12).Signals(2).Name = 'state_VBattery'
      | sbobj.Groups(12).Signals(2).XData = [0 100]
      | sbobj.Groups(12).Signals(2).YData = [10 10]
      | sbobj.Groups(12).Signals(3).Name = 'flt_HOT'
      | sbobj.Groups(12).Signals(3).XData = [0 100]
      | sbobj.Groups(12).Signals(3).YData = [50 50]
      | sbobj.Groups(12).Signals(4).Name = 'flt_ECT'
      | sbobj.Groups(12).Signals(4).XData = [0 100]
      | sbobj.Groups(12).Signals(4).YData = [40 40]
      | sbobj.Groups(12).Signals(5).Name = 'dfbk_GlowPlugOutput'
      | sbobj.Groups(12).Signals(5).XData = [0 0.8 0.8 10.6 10.6 14.6 66 67 67 75.6 75.6 100]
      | sbobj.Groups(12).Signals(5).YData = [0 0 1 1 0 0 0 0 1 1 0 0]
      | sbobj.Groups(12).Signals(6).Name = 'din_GlowPlugRelay'
      | sbobj.Groups(12).Signals(6).XData = [0 0.8 0.8 10.8 10.8 14.6 66 67 67 75.5 75.5 100]
      | sbobj.Groups(12).Signals(6).YData = [0 0 1 1 0 0 0 0 1 1 0 0]
      | sbobj.Groups(12).Signals(7).Name = 'state_System'
      | sbobj.Groups(12).Signals(7).XData = [0 1.7 1.7 10.7 10.7 14.5 14.5 68.5 68.5 69.8 69.8 75.6 75.6 77.5 77.5 100]
      | sbobj.Groups(12).Signals(7).YData = [3 3 1 1 3 3 1 1 3 3 1 1 3 3 1 1]
      | sbobj.Groups(12).Signals(8).Name = 'dout_GlowPlug'
      | sbobj.Groups(12).Signals(8).XData = [0 1.7 1.7 10.7 10.7 67 67 68.5 68.5 71.1 71.1 75.6 75.6 100]
      | sbobj.Groups(12).Signals(8).YData = [0 0 1 1 0 0 1 1 0 0 1 1 0 0]
      | sbobj.Groups(12).Signals(9).Name = 'state_GlowPlugOutput'
      | sbobj.Groups(12).Signals(9).XData = [0 100]
      | sbobj.Groups(12).Signals(9).YData = [8 8]
      | sbobj.Groups(12).Signals(10).Name = 'state_GlowPlugRelay'
      | sbobj.Groups(12).Signals(10).XData = [0 100]
      | sbobj.Groups(12).Signals(10).YData = [8 8]
      | sbobj.Groups(13).Name = 'T13-Voltage'
      | sbobj.Groups(13).Signals(1).Name = 'state_Engine'
      | sbobj.Groups(13).Signals(1).XData = [0 67 67 100]
      | sbobj.Groups(13).Signals(1).YData = [1 1 2 2]
      | sbobj.Groups(13).Signals(2).Name = 'state_VBattery'
      | sbobj.Groups(13).Signals(2).XData = [0 0.4 0.4 35.9 35.9 40 40 44.1 44.1 69.1 69.1 70.8 70.8 100]
      | sbobj.Groups(13).Signals(2).YData = [8 8 22 22 9 9 10.5 10.5 8 8 22 22 8 8]
      | sbobj.Groups(13).Signals(3).Name = 'flt_HOT'
      | sbobj.Groups(13).Signals(3).XData = [0 100]
      | sbobj.Groups(13).Signals(3).YData = [50 50]
      | sbobj.Groups(13).Signals(4).Name = 'flt_ECT'
      | sbobj.Groups(13).Signals(4).XData = [0 100]
      | sbobj.Groups(13).Signals(4).YData = [40 40]
      | sbobj.Groups(13).Signals(5).Name = 'dfbk_GlowPlugOutput'
      | sbobj.Groups(13).Signals(5).XData = [0 40.1 40.1 66.6 66.6 67 67 68.7 68.7 100]
      | sbobj.Groups(13).Signals(5).YData = [0 0 1 1 0 0 1 1 0 0]
      | sbobj.Groups(13).Signals(6).Name = 'din_GlowPlugRelay'
      | sbobj.Groups(13).Signals(6).XData = [0 40 40 66 66 67.1 67.1 68.7 68.7 100]
      | sbobj.Groups(13).Signals(6).YData = [0 0 1 1 0 0 1 1 0 0]
      | sbobj.Groups(13).Signals(7).Name = 'state_System'
      | sbobj.Groups(13).Signals(7).XData = [0 77.5 100]
      | sbobj.Groups(13).Signals(7).YData = [1 1 1]
      | sbobj.Groups(13).Signals(8).Name = 'dout_GlowPlug'
      | sbobj.Groups(13).Signals(8).XData = [0 40 40 67 67 67.1 67.1 69.1 69.1 100]
      | sbobj.Groups(13).Signals(8).YData = [0 0 1 1 0 0 1 1 0 0]
      | sbobj.Groups(13).Signals(9).Name = 'state_GlowPlugOutput'
      | sbobj.Groups(13).Signals(9).XData = [0 100]
      | sbobj.Groups(13).Signals(9).YData = [8 8]
      | sbobj.Groups(13).Signals(10).Name = 'state_GlowPlugRelay'
      | sbobj.Groups(13).Signals(10).XData = [0 100]
      | sbobj.Groups(13).Signals(10).YData = [8 8]
      | sbobj.Groups(14).Name = 'T14-Voltage2'
      | sbobj.Groups(14).Signals(1).Name = 'state_Engine'
      | sbobj.Groups(14).Signals(1).XData = [0 67 67 100]
      | sbobj.Groups(14).Signals(1).YData = [1 1 2 2]
      | sbobj.Groups(14).Signals(2).Name = 'state_VBattery'
      | sbobj.Groups(14).Signals(2).XData = [0 0.4 0.4 20 20 30 30 100]
      | sbobj.Groups(14).Signals(2).YData = [8 8 22 22 8 8 22 22]
      | sbobj.Groups(14).Signals(3).Name = 'flt_HOT'
      | sbobj.Groups(14).Signals(3).XData = [0 100]
      | sbobj.Groups(14).Signals(3).YData = [50 50]
      | sbobj.Groups(14).Signals(4).Name = 'flt_ECT'
      | sbobj.Groups(14).Signals(4).XData = [0 100]
      | sbobj.Groups(14).Signals(4).YData = [40 40]
      | sbobj.Groups(14).Signals(5).Name = 'dfbk_GlowPlugOutput'
      | sbobj.Groups(14).Signals(5).XData = [0 20.2 20.2 30 30 100]
      | sbobj.Groups(14).Signals(5).YData = [0 0 1 1 0 0]
      | sbobj.Groups(14).Signals(6).Name = 'din_GlowPlugRelay'
      | sbobj.Groups(14).Signals(6).XData = [0 20 20 30 30 100]
      | sbobj.Groups(14).Signals(6).YData = [0 0 1 1 0 0]
      | sbobj.Groups(14).Signals(7).Name = 'state_System'
      | sbobj.Groups(14).Signals(7).XData = [0 77.5 100]
      | sbobj.Groups(14).Signals(7).YData = [1 1 1]
      | sbobj.Groups(14).Signals(8).Name = 'dout_GlowPlug'
      | sbobj.Groups(14).Signals(8).XData = [0 20 20 30 30 100]
      | sbobj.Groups(14).Signals(8).YData = [0 0 1 1 0 0]
      | sbobj.Groups(14).Signals(9).Name = 'state_GlowPlugOutput'
      | sbobj.Groups(14).Signals(9).XData = [0 100]
      | sbobj.Groups(14).Signals(9).YData = [8 8]
      | sbobj.Groups(14).Signals(10).Name = 'state_GlowPlugRelay'
      | sbobj.Groups(14).Signals(10).XData = [0 100]
      | sbobj.Groups(14).Signals(10).YData = [8 8]
      | sbobj.Groups(15).Name = 'T15-ErrorOn'
      | sbobj.Groups(15).Signals(1).Name = 'state_Engine'
      | sbobj.Groups(15).Signals(1).XData = [0 100]
      | sbobj.Groups(15).Signals(1).YData = [1 1]
      | sbobj.Groups(15).Signals(2).Name = 'state_VBattery'
      | sbobj.Groups(15).Signals(2).XData = [0 100]
      | sbobj.Groups(15).Signals(2).YData = [8 8]
      | sbobj.Groups(15).Signals(3).Name = 'flt_HOT'
      | sbobj.Groups(15).Signals(3).XData = [0 100]
      | sbobj.Groups(15).Signals(3).YData = [140 140]
      | sbobj.Groups(15).Signals(4).Name = 'flt_ECT'
      | sbobj.Groups(15).Signals(4).XData = [0 100]
      | sbobj.Groups(15).Signals(4).YData = [40 40]
      | sbobj.Groups(15).Signals(5).Name = 'dfbk_GlowPlugOutput'
      | sbobj.Groups(15).Signals(5).XData = [0 74.4 74.4 100]
      | sbobj.Groups(15).Signals(5).YData = [0 0 1 1]
      | sbobj.Groups(15).Signals(6).Name = 'din_GlowPlugRelay'
      | sbobj.Groups(15).Signals(6).XData = [0 44.2 44.2 74.4 74.4 100]
      | sbobj.Groups(15).Signals(6).YData = [1 1 0 0 1 1]
      | sbobj.Groups(15).Signals(7).Name = 'state_System'
      | sbobj.Groups(15).Signals(7).XData = [0 30.5 30.5 100]
      | sbobj.Groups(15).Signals(7).YData = [0 0 1 1]
      | sbobj.Groups(15).Signals(8).Name = 'dout_GlowPlug'
      | sbobj.Groups(15).Signals(8).XData = [0 59.4 59.4 64.7 64.7 100]
      | sbobj.Groups(15).Signals(8).YData = [0 0 1 1 0 0]
      | sbobj.Groups(15).Signals(9).Name = 'state_GlowPlugOutput'
      | sbobj.Groups(15).Signals(9).XData = [0 64.6 64.6 100]
      | sbobj.Groups(15).Signals(9).YData = [8 8 3 3]
      | sbobj.Groups(15).Signals(10).Name = 'state_GlowPlugRelay'
      | sbobj.Groups(15).Signals(10).XData = [0 30.2 30.2 59.3 59.3 100]
      | sbobj.Groups(15).Signals(10).YData = [8 8 2 2 8 8]
  state_Engine : Outport  Tag=STV Outport
  state_VBattery : Outport  Tag=STV Outport  Port=2
  flt_HOT : Outport  Tag=STV Outport  Port=3
  flt_ECT : Outport  Tag=STV Outport  Port=4
  dfbk_GlowPlugOutput : Outport  Tag=STV Outport  Port=5
  din_GlowPlugRelay : Outport  Tag=STV Outport  Port=6
  state_System : Outport  Tag=STV Outport  Port=7
  dout_GlowPlug : Outport  Tag=STV Outport  Port=8
  state_GlowPlugOutput : Outport  Tag=STV Outport  Port=9
  state_GlowPlugRelay : Outport  Tag=STV Outport  Port=10
  wires:
  Demux/1 -> state_Engine/1
  FromWs/1 -> Demux/1
  Demux/2 -> state_VBattery/1
  Demux/3 -> flt_HOT/1
  Demux/4 -> flt_ECT/1
  Demux/5 -> dfbk_GlowPlugOutput/1
  Demux/6 -> din_GlowPlugRelay/1
  Demux/7 -> state_System/1
  Demux/8 -> dout_GlowPlug/1
  Demux/9 -> state_GlowPlugOutput/1
  Demux/10 -> state_GlowPlugRelay/1

== stateflow chart GlowPlug/GlowPlug ==
  state INACTIVE
    en:dout_GlowPlug = INACTIVE;
    en:count_GlowPlug = 0;
    state RESET_CRANK
      en:state_CrankTimerExpired = INACTIVE;
    state CRANKING
    CRANKING -> RESET_CRANK : [(state_Engine != ENGINE_CRANKING)...
        | && (CD_GLOW_PLUG_CRANKING_FUNCTION != NON_FUNCTIONAL)]
    (default) -> CRANKING
  state AFTERGLOW
    en:dout_GlowPlug = ACTIVE;
    du:debounceCount--;
    ex:glowPlugAfterGlowDone = ACTIVE;
    en:count_GlowPlug = 0;
  state GLOW_DURING_CRANK
    en:dout_GlowPlug = ACTIVE;
    en:debounceCrank = 0;
    du:debounceCrank++;
    ex:state_CrankTimerExpired = ACTIVE;
    en:glowPlugAfterGlowDone = INACTIVE;
  state WAIT_STARTUP
    en:dout_GlowPlug = 0;
    en:debounceCrank = 0;
    du:debounceCrank++;
  note: // Wait X amout of time to make sure we have a stead temperature reading.
  state PreheatTime(temp) [function]
    (junction 26) -> (junction 31) : {debounceCount = CD_GLOW_PLUG_PREHEAT_TIME_LEVEL0;}
    (junction 30) -> (junction 27) : {debounceCount = CD_GLOW_PLUG_PREHEAT_TIME_LEVEL1;}
    (junction 25) -> (junction 30) [order 1] : [temp < CD_GLOW_PLUG_TEMP_LEVEL2]
    (junction 32) -> (junction 28) [order 2] : {debounceCount = CD_GLOW_PLUG_PREHEAT_TIME_LEVEL3;}
    (junction 17) -> (junction 28)
    (junction 33) -> (junction 17) : {debounceCount = CD_GLOW_PLUG_PREHEAT_TIME_LEVEL2;}
    (junction 32) -> (junction 33) [order 1] : [temp < CD_GLOW_PLUG_TEMP_LEVEL3]
    (junction 31) -> (junction 27)
    (default) -> (junction 24) : /* Glow plug preheat time */
    (junction 24) -> (junction 25) [order 2]
    (junction 24) -> (junction 26) [order 1] : [temp < CD_GLOW_PLUG_TEMP_LEVEL1]
    (junction 28) -> (junction 29)
    (junction 25) -> (junction 32) [order 2]
    (junction 27) -> (junction 17)
  state PreheatWaitTime(temp) [function]
    (default) -> (junction 35) : /* Glow plug preheat time */
    (junction 35) -> (junction 36) [order 1] : [temp < CD_GLOW_PLUG_TEMP_LEVEL1]
    (junction 35) -> (junction 37) [order 2]
    (junction 36) -> (junction 44) : {debounceCount = CD_GLOW_PLUG_WAIT_TIME_LEVEL0;}
    (junction 37) -> (junction 38) [order 1] : [temp < CD_GLOW_PLUG_TEMP_LEVEL2]
    (junction 37) -> (junction 39) [order 2]
    (junction 38) -> (junction 43) : {debounceCount = CD_GLOW_PLUG_WAIT_TIME_LEVEL1;}
    (junction 39) -> (junction 40) [order 1] : [temp < CD_GLOW_PLUG_TEMP_LEVEL3]
    (junction 39) -> (junction 41) [order 2] : {debounceCount = CD_GLOW_PLUG_WAIT_TIME_LEVEL3;}
    (junction 40) -> (junction 42) : {debounceCount = CD_GLOW_PLUG_WAIT_TIME_LEVEL2;}
    (junction 42) -> (junction 41)
    (junction 43) -> (junction 42)
    (junction 44) -> (junction 43)
    (junction 41) -> (junction 45)
  state AfterglowTime(temp) [function]
    (junction 50) -> (junction 52) [order 2] : {debounceCount = CD_GLOW_PLUG_AFTERGLOW_TIME_LEVEL3;}
    (junction 52) -> (junction 19)
    (junction 18) -> (junction 34)
    (junction 51) -> (junction 53) : {debounceCount = CD_GLOW_PLUG_AFTERGLOW_TIME_LEVEL2;}
    (junction 53) -> (junction 52)
    (junction 34) -> (junction 53)
    (junction 50) -> (junction 51) [order 1] : [temp < CD_GLOW_PLUG_TEMP_LEVEL3]
    (junction 49) -> (junction 34) : {debounceCount = CD_GLOW_PLUG_AFTERGLOW_TIME_LEVEL1;}
    (default) -> (junction 46) : /* Glow plug preheat time */
    (junction 46) -> (junction 47) [order 1] : [temp < CD_GLOW_PLUG_TEMP_LEVEL1]
    (junction 46) -> (junction 48) [order 2]
    (junction 47) -> (junction 18) : {debounceCount = CD_GLOW_PLUG_AFTERGLOW_TIME_LEVEL0;}
    (junction 48) -> (junction 49) [order 1] : [temp < CD_GLOW_PLUG_TEMP_LEVEL2]
    (junction 48) -> (junction 50) [order 2]
  state PREHEAT
    state PREGLOW_WAIT
      en:dout_GlowPlug = INACTIVE;
      en:cycleCount++;
      du:debounceCount--;
    state PREGLOW
      du:debounceCount--;
      du:count_GlowPlug = debounceCount;
      note: We only want the output active if the count is greater than zero.  If it equals zero we want to have
          | the output off.  That way when we enter the loop and the counter is set to zero the glow plugs
          | will not flash on for 1 count.
      (default) -> (junction 20)
      (junction 20) -> (junction 21) [order 1] : [(debounceCount != 0)]
      (junction 21) -> (junction 23) : {
          | dout_GlowPlug = ACTIVE;
          | }
      (junction 23) -> (junction 22)
      (junction 20) -> (junction 22) [order 2] : {
          | dout_GlowPlug = INACTIVE;
          | }
    PREGLOW -> PREGLOW_WAIT : [(debounceCount == 0)]
        | {
        | PreheatWaitTime(MachineTemp);
        | }
    PREGLOW_WAIT -> PREGLOW : [(debounceCount == 0)]
        | {
        | PreheatTime(MachineTemp);
        | }
    (default) -> PREGLOW
  INACTIVE -> PREHEAT [order 3] : [(CD_GLOW_PLUG_PREHEAT_FUNCTION != NON_FUNCTIONAL)...
      | && (cycleCount < CD_GLOW_PLUG_PREHEAT_COUNTER)...
      | && (state_VBattery != OORL)...
      | && ((CD_GLOW_PLUG_OFF_WITH_LOW_BATTERY == NON_FUNCTIONAL) || (state_VBattery == NORMAL) || (state_VBattery == HIGH))...
      | && ((state_GlowPlugOutput == NORMAL) || (state_GlowPlugOutput == FAILURE))...
      | && (state_GlowPlugRelay == NORMAL)...
      | && (state_Engine == ENGINE_NOT_RUNNING)...
      | && (state_System == SYS_NORMAL)]
      | {
      | PreheatTime(MachineTemp);
      | }
  INACTIVE -> AFTERGLOW [order 1] : [(CD_GLOW_PLUG_AFTERGLOW_FUNCTION != NON_FUNCTIONAL)...
      | && (state_Engine == ENGINE_RUNNING)...
      | && ((state_GlowPlugOutput == NORMAL) || (state_GlowPlugOutput == FAILURE))...
      | && (state_GlowPlugRelay == NORMAL)...
      | && (glowPlugAfterGlowDone == INACTIVE)]
      | {
      | AfterglowTime(MachineTemp);
      | }
  AFTERGLOW -> INACTIVE : [(debounceCount == 0)...
      | || !((state_GlowPlugOutput == NORMAL) || (state_GlowPlugOutput == FAILURE))...
      | || (state_GlowPlugRelay != NORMAL)...
      | || (state_System != SYS_NORMAL)]
  PREHEAT -> INACTIVE : [(state_Engine == ENGINE_RUNNING)...
      | || (state_Engine == ENGINE_CRANKING)...
      | || !((state_GlowPlugOutput == NORMAL) || (state_GlowPlugOutput == FAILURE))...
      | || (state_GlowPlugRelay != NORMAL)...
      | || (state_System != SYS_NORMAL)...
      | || (state_VBattery == OORL)...
      | || (cycleCount >= CD_GLOW_PLUG_PREHEAT_COUNTER)]
      | {
      | cycleCount = CD_GLOW_PLUG_PREHEAT_COUNTER;
      | }
  WAIT_STARTUP -> INACTIVE : [(debounceCrank > 3)]
  GLOW_DURING_CRANK -> INACTIVE : [(state_Engine != ENGINE_CRANKING)...
      | || !((state_GlowPlugOutput == NORMAL) || (state_GlowPlugOutput == FAILURE))...
      | || (state_GlowPlugRelay != NORMAL)...
      | || (state_VBattery == OORL)...
      | || (state_System != SYS_NORMAL)...
      | || ((debounceCrank >= CD_GLOW_PLUG_DEBOUNCE_CRANK)...
      |    && (CD_GLOW_PLUG_DEBOUNCE_CRANK != UNLIMITED))]
  INACTIVE -> GLOW_DURING_CRANK [order 2] : [(CD_GLOW_PLUG_CRANKING_FUNCTION != NON_FUNCTIONAL)...
      | && (state_VBattery != OORL)...
      | && (state_Engine == ENGINE_CRANKING)...
      | && ((state_GlowPlugOutput == NORMAL) || (state_GlowPlugOutput == FAILURE))...
      | && (state_GlowPlugRelay == NORMAL)...
      | && (state_CrankTimerExpired != ACTIVE)]
  (default) -> WAIT_STARTUP
  data: temp function_input uint16; temp function_input uint16; temp function_input uint16; state_Engine input uint8; state_VBattery input uint8; MachineTemp input uint16; dout_GlowPlug output boolean; state_GlowPlugOutput input uint8; state_GlowPlugRelay input uint8; CD_GLOW_PLUG_PREHEAT_FUNCTION parameter uint8; CD_GLOW_PLUG_TEMP_LEVEL1 parameter uint16; CD_GLOW_PLUG_PREHEAT_TIME_LEVEL0 parameter uint16; CD_GLOW_PLUG_TEMP_LEVEL2 parameter uint16; CD_GLOW_PLUG_TEMP_LEVEL3 parameter uint16; CD_GLOW_PLUG_WAIT_TIME_LEVEL1 parameter uint16; CD_GLOW_PLUG_PREHEAT_TIME_LEVEL2 parameter uint16; CD_GLOW_PLUG_PREHEAT_TIME_LEVEL3 parameter uint16; CD_GLOW_PLUG_WAIT_TIME_LEVEL2 parameter uint16; CD_GLOW_PLUG_WAIT_TIME_LEVEL3 parameter uint16; CD_GLOW_PLUG_WAIT_TIME_LEVEL0 parameter uint16; CD_GLOW_PLUG_PREHEAT_TIME_LEVEL1 parameter uint16; CD_GLOW_PLUG_AFTERGLOW_FUNCTION parameter uint8; CD_GLOW_PLUG_AFTERGLOW_TIME_LEVEL0 parameter uint16; CD_GLOW_PLUG_AFTERGLOW_TIME_LEVEL1 parameter uint16; CD_GLOW_PLUG_AFTERGLOW_TIME_LEVEL2 parameter uint16; CD_GLOW_PLUG_AFTERGLOW_TIME_LEVEL3 parameter uint16; CD_GLOW_PLUG_CRANKING_FUNCTION parameter uint8; CD_GLOW_PLUG_OFF_WITH_LOW_BATTERY parameter uint8; debounceCount local uint16 =0; cycleCount local uint16 =0; glowPlugAfterGlowDone local boolean =0; CD_GLOW_PLUG_PREHEAT_COUNTER parameter uint8; count_GlowPlug output uint16; ENGINE_CRANKING parameter uint8 =2; ENGINE_NOT_RUNNING parameter uint8 =1; ENGINE_RUNNING parameter uint8 =3; NORMAL parameter uint8 =8; ACTIVE parameter uint8 =1; INACTIVE parameter uint8 =0; state_System input uint8; SYS_NORMAL parameter uint8; HIGH parameter uint8; state_CrankTimerExpired local uint8; debounceCrank local uint16 =0; CD_GLOW_PLUG_DEBOUNCE_CRANK parameter uint16; UNLIMITED parameter uint16; NON_FUNCTIONAL parameter uint8; OORL parameter uint8; FAILURE parameter uint8
  data cycleCount settings: description=Counts the number of cycles the glow plugs are active.
  data count_GlowPlug settings: description=Used to output counter to panel.
